simulink model "power_FCHPS_MEA2"  (R2017b)
settings: Solver=ode23tb  StartTime=0.0  StopTime=350  RelTol=1e-3  EnableMultiTasking=on
PreLoadFcn:
  | Ts=100e-6;
InitFcn:
  | Ts=100e-6;
undefined symbols (not defined in the file): DiscIntNeverNeededParam, Ion, Lithium
libraries: powerlib x94, simulink x8, powerlib_meascontrol x3, electricdrivelib x3
(part 1 of 4)
settings Model: SimulationMode=accelerator  Creator=MathWorks  LastModifiedBy=vv
settings DataIOCC: LimitDataPoints=on  SaveFormat=Array  SignalLoggingSaveFormat=ModelDataLogs
settings OptimizationCC: ExpressionDepthLimit=2147483647  EfficientMapNaN2IntZero=off  LifeSpan=inf
settings DebuggingCC: UnderspecifiedInitializationDetection=Classic  MergeDetectMultiDrivingBlocksExec=none  SolverPrmCheckMsg=warning  FcnCallInpInsideContextMsg=warning  AllowSymbolicDim=off  StateNameClashWarn=warning  SFUnexpectedBacktrackingDiag=warning  SFNoUnconditionalDefaultTransitionDiag=warning  SFExecutionAtInitializationDiag=none
settings HardwareCC: ProdBitPerPointer=32  ProdBitPerSizeT=32  ProdBitPerPtrDiffT=32  ProdLargestAtomicFloat=None  ProdIntDivRoundTo=Undefined  ProdEndianess=Unspecified  ProdWordSize=32  ProdHWDeviceType=32-bit Generic  TargetBitPerPointer=64  TargetBitPerSizeT=64  TargetBitPerPtrDiffT=64  TargetLongLongMode=on  TargetIntDivRoundTo=Zero  TargetEndianess=LittleEndian  TargetWordSize=64  TargetHWDeviceType=MATLAB Host  ProdEqTarget=off
settings ModelReferenceCC: PropagateSignalLabelsOutOfModel=off
settings CodeAppCC: MaxIdLength=128  StateflowObjectComments=on
settings GRTTargetCC: TargetLangStandard=C89/C90 (ANSI)  CombineOutputUpdateFcns=off  GRTInterface=on
settings ConfigComp: CovMetricSettings=dw  CovHtmlReporting=on  CovSaveCumulativeToWorkspaceVar=on  CovSaveSingleToWorkspaceVar=on  CovExternalEMLEnable=off  CovSFcnEnable=off
settings SimscapeCC: SimscapeNormalizeSystem=off

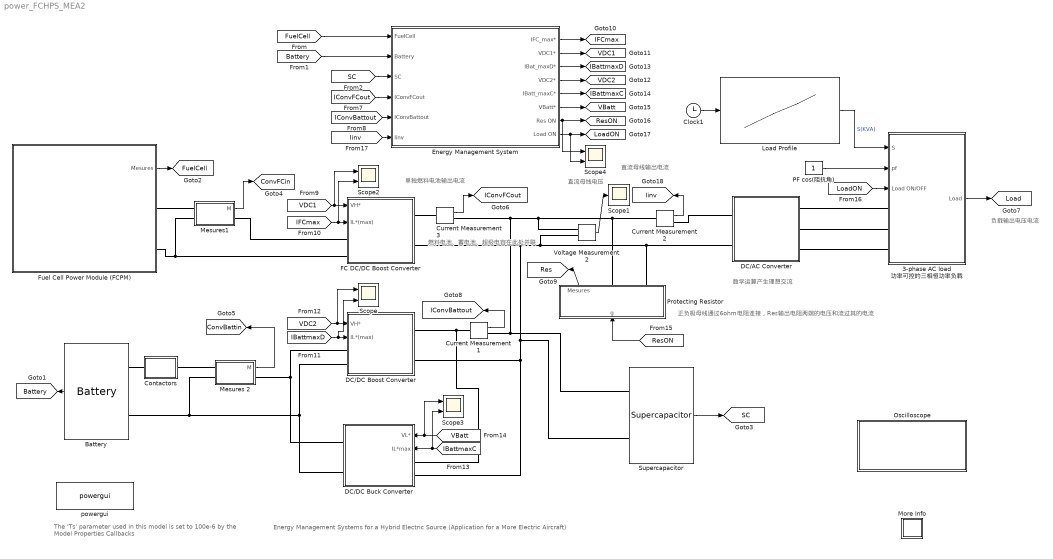
== system power_FCHPS_MEA2 ==
  note: 直流母线电压
  note: 直流母线输出电流
  note: 单独燃料电池输出电流
  note: 燃料电池、蓄电池、超级电容在此处并联
  note: 正负极母线通过6ohm电阻连接，Res输出电阻两端的电压和流过其的电流
  note: 数学运算产生理想交流
  note: 负载输出电压电流
  note: Energy Management Systems for a Hybrid Electric Source (Application for a More Electric Aircraft)
  note: The 'Ts' parameter used in this model
      | is set to 100e-6  by the Model Properties Callbacks
  3-phase AC load 功率可控的三相恒功率负载 : Subsystem
      mask Display: image(imread('load.png'))
  Battery : electricdrivelib/Extra Sources/Battery  BatType=Lithium-Ion  ShowTempParam=off  ThermalPreset=no  ShowAgeParam=off  NomV=48  NomQ=40  SOC=65  Batt_Tr=20  PresetModel=off  MaxQ=40  MinV=36  FullV=55.8714  Dis_rate=17.3913  R=0.012  Normal_OP=36.1739  expZone="[52.3         1.96]"  current=[20 80]  Units=Ampere-hour  Tci=20  NomT=20  T2=-30  MaxQ2=4.8  FullV2=7.1  Normal_OP2=5.72  expZone2="[6.58  1]"  Rca=0.6  ti=1000  Dp=0  Neq0=0  Tsim=1e6  Ta1=25  Qeol=5.4*0.9  Reol=0.013333*1.2  Char_age=[2.3478, 3]  Dis_age=[2.3478, 10]  N1=1500  N2=10500  N3=1000  N4=1400  Ta2=45  N5=950
  Clock1 : Clock
  Contactors : Subsystem
  Current Measurement1 : powerlib/Measurements/Current Measurement  PhasorSimulation=off  OutputType=Complex  PSBequivalent=0
  Current Measurement2 : powerlib/Measurements/Current Measurement  PhasorSimulation=off  OutputType=Complex  PSBequivalent=0
  Current Measurement3 : powerlib/Measurements/Current Measurement  PhasorSimulation=off  OutputType=Complex  PSBequivalent=0
  DC/AC Converter : Subsystem  mask(Average-value Inverter model){VL=200, f=400, n=97}
      mask prompts: VL "Output Line Voltage (Vrms)"; f "Output frequency (Hz)"; n "Nominal Efficiency (%)"
      mask help: This block represents an average-value inverter model which includes the converter efficiency.
      mask Display: image(imread('DCAC.bmp'))
  DC/DC Boost Converter : Subsystem  mask(Average value DC/DC boost converter){Inom=18, n=[80 88], Tr=0.1, CL=15.6}
      mask prompts: Inom "Full load current (A)"; n "Efficiency @ Full and 10% load  (%) [n1, n2]"; Tr "Response time (s) (Voltage Regulator)"; CL "Load Capacitance (F)"
      mask help: This block implements an average-value DC/DC boost converter. Two inputs are provided for output voltage regulation and input current limitation
      mask Display: image(imread('DCDC.bmp'))
  DC/DC Buck Converter : Subsystem  mask(Average Value Buck DC/DC Converter){Inom=20, n=[80 88], Tr=0.1, CL=100e-3}
      mask prompts: Inom "Full load current (A)"; n "Efficiency @ Full and 10% load (%) [n1, n2]"; Tr "Response Time (s) (Voltage Regulator)"; CL "Load Capacitance (F)"
      mask help: This block implements an average-value DC/DC buck converter. Two inputs are provided for output voltage regulation and output current limitation
      mask init:
      | L=10e-3; C=800e-6+CL;
      | thau_s=Tr;  %response time
      | %Current regulator
      | zetai=0.995;
      | thau_si=0.1/10; 
      | %zetawni=4.6/thau_si;
      | zetawni=(-log(0.05*sqrt(1-zetai^2)))/thau_si;
      | Kpi=2*L*zetawni;
      | wni=zetawni/zetai;
      | Kii=L*wni^2;
      | %Voltage regulator
      | zetav=0.995;
      | thau_sv=thau_s; %response time
      | %zetawnv=4.6/thau_sv;
      | zetawnv=(-log(0.05*sqrt(1-zetav^2)))/thau_sv;
      | Kpv=2*C*zetawnv;
      | wnv=zetawnv/zetav;
      | Kiv=C*wnv^2;
      | k=((n(1)/100)-(n(2)/100))/(Inom-(0.1*Inom));
      | k0=(n(1)/100)-k*Inom;
      mask DialogControl ParameterTabVar0 Prompt: Parameters
      mask Display: image(imread('DCDC.bmp'))
  Energy Management System : Subsystem  mask(Energy Management System){ems=State Machine Control Strategy}
      mask prompts: ems "Strategy:"
      mask help:
      | This block implements six types of energy management strategies, commonly used in Fuel Cell Hybrid Power Systems
      |
      | The ECMS and EEMS Control Strategies require the Optimization toolbox. The State Machine Control Strategy is selected automatically when the toolbox is not available.
      mask init:
      | [X1,X1m,X2,X2m,X3,X4,Y1,Y1m,Y2,Y2m,Y3,Y4,color1,color2]=spsdrivelogo;
      | 
      | SimulinkModel  = [gcs,'/Energy Management System'];
      | SimulinkModel2 = [gcs,'/Energy Management System/Model'];
      | 
      | switch ems
      |     case 'State Machine Control Strategy'
      |         set_param(SimulinkModel2,'OverrideUsingVariant','FrequencyDecoupling');
      |         
      |     case 'Classical PI Control Strategy'
      |         set_param(SimulinkModel2,'OverrideUsingVariant','ClassicalPI');
      |         
      |     case 'Rule Based Fuzzy Logic Control Strategy'
      |         if isempty(ver('fuzzy'))
      |             set_param(SimulinkModel,'ems','State Machine Control Strategy');
      |             set_param(SimulinkModel2,'OverrideUsingVariant','FrequencyDecoupling');
      |         else
      |             fuzzy_control=READFIS('fuzzy control.fis');
      |             set_param(SimulinkModel2,'OverrideUsingVariant','RuleBasedFuzzyLogic');
      |         end
      |         
      |     case 'Frequency Decoupling and State Machine Control Strategy'
      |         set_param(SimulinkModel2,'OverrideUsingVariant','FrequencyDecoupling');
      | 
      |     case 'Equivalent Consumption Minimization Strategy (ECMS)'
      |         if isempty(ver('optim'))
      |             set_param(SimulinkModel,'ems','State Machine Control Strategy');
      |             set_param(SimulinkModel2,'OverrideUsingVariant','FrequencyDecoupling');
      |         else
      |             set_param(SimulinkModel2,'OverrideUsingVariant','ECMS');
      |         end
      |         
      |     case 'External Energy Maximization Strategy (EEMS)'
      |         if isempty(ver('optim'))
      |             set_param(SimulinkModel,'ems','State Machine Control Strategy');
      |             set_param(SimulinkModel2,'OverrideUsingVariant','FrequencyDecoupling');
      |         else
      |             set_param(SimulinkModel2,'OverrideUsingVariant','EEMS');
      |         end
      | end
      mask TypeOptions ems: State Machine Control Strategy | Classical PI Control Strategy | Frequency Decoupling and State Machine Control Strategy | Equivalent Consumption Minimization Strategy (ECMS) | External Energy Maximization Strategy (EEMS)
      mask Display:
      | patch([X1 X1m],[Y1 Y1m],color1);
      | patch(X3,Y3,color2);
      | plot([X1 X1m X2 X2m X3 X4],[Y1 Y1m Y2 Y2m Y3 Y4]);
  FC DC/DC Boost Converter : Subsystem  mask(Average value DC/DC boost converter){Inom=45, n=[85 90], Tr=0.1, CL=15.6}
      mask prompts: Inom "Full load current (A)"; n "Efficiency @ Full and 10% load  (%) [n1, n2]"; Tr "Response time (s) (Voltage Regulator)"; CL "Load Capacitance (F)"
      mask help: This block implements an average-value DC/DC boost converter. Two inputs are provided for output voltage regulation and input current limitation
      mask Display: image(imread('DCDC.bmp'))
  Fuel Cell Power Module (FCPM) : Subsystem
      mask Display: image(imread('power_stack.bmp'))
  Load Profile : Lookup_n-D  NumberOfTableDimensions=1  BreakpointsForDimension1="[0    20    30    35    40    45    50    60    70    90   125   130   140   160   170   180   190 210   220   230   235   245   250   260   270   300   310   320   330   340     350]"  BreakpointsForDimension2=[0 571.55 685.8 800.15 914.4 1028.8 1143.1 1257.4 1371.7 1486 1600.3 1714.6 1828.9 1943.2 2057.5 2171.8 2286.1 2400.5 2514.7 2629.1 2743.3 2857.7 2971.9 3086.3 3200.5 3314.9 3429.2]  Table="[0         0         0         0         0    5.8000    4.8000    4.8000   10.0000    9.4000  10.5000    5.0000    8.8000    7.0000    7.3000    2.5000    8.5000    7.5000    9.0000    8.9000 8.7000    0.7000    2.9000    2.3500    2.9000    2.9000    2.4000    2.9000    2.9000         0     0]"  InternalRulePriority=Speed  RndMeth=Simplest  InputSameDT=on
  Mesures 2 : Subsystem
  Mesures1 : Subsystem
  More Info : Subsystem
      settings: OpenFcn=showdemo(bdroot(gcb))
      mask Display: disp('?')
  Oscilloscope : Subsystem
      mask Display: color('blue');disp('Measurements')
  PF cos(阻抗角) : Constant
  Protecting Resistor : Subsystem
      mask Display: image(imread('Res.jpg'))
  Scope{,2..4} (4 alike) : Scope  NumInputPorts=2
  Scope1 : Scope
  Supercapacitor : electricdrivelib/Extra Sources/Supercapacitor  C=15.6  Rdc=150e-3  Voltage=291.6  Ns=108  Np=1  Vinit=270  Temp=25  PresetModel=on  EstParam=off  Nc=1  r=1e-9  epsilon=6.0208e-10  Ich=10  Vstern="[0.161  2.7  7.8]"  Self_dis=on  Ioc=10  Vself="[48  47.8  47.06  44.65]"  demandeplot=off  I="[10  20 100  500]"  Units=sec  Vmax=0  If=0  deltaV=0.3  alpha=0.3  sec=0
      settings: SourceProductName=Simscape Power Systems  SourceProductBaseCode=PS
  Voltage Measurement2 : powerlib/Measurements/Voltage Measurement  PhasorSimulation=off  OutputType=Complex  PSBequivalent=0
  powergui : powerlib/powergui  Priority=1  SimulationMode=Discrete  SampleTime=Ts  frequency=60  Iterations=50  frequencyindice=0  Pbase=100e6  ErrMax=1e-4  UnitsV=kV  UnitsW=MW  buscounter=0  FunctionMessages=off  echomessages=off  EnableUseOfTLC=off  CurrentSourceSwitches=off  DisableSnubberDevices=off  DisableRonSwitches=off  DisableVfSwitches=off  DisplayEquations=off  SolverType=Tustin/Backward Euler (TBE)  Interpol=off  ExternalGateDelay=off  methode=off  Ts=0  x0status=blocks  SPID=off  SwTol=0  HookPort=off  RestoreLinks=warning  ResistiveCurrentMeasurement=off  Frange=[0:2:500]  Ylog=off  Xlog=on  ShowGrid=off  save=off  variable=ZData  structure=0  ZoomFFT=off  StartTime=0.0  cycles=1  DisplayStyle=1  fundamental=60  FreqAxis=off  MaxFrequency=1000  frequencyindicesteady=1  RmsSteady=1  display=off
  tag scope: Battery=global, ConvBattin=global, ConvFCin=global, FuelCell=global, IBattmaxC=global, IBattmaxD=global, IConvBattout=global, IConvFCout=global, IFCmax=global, Iinv=global, Load=global, LoadON=global, Res=global, ResON=global, SC=global, VBatt=global, VDC1=global, VDC2=global
  wires:
  Fuel Cell Power Module (FCPM)/1(Mesures) -> [FuelCell]
  Mesures1/1(M) -> [ConvFCin]
  Current Measurement1/1 -> [IConvBattout]
  Current Measurement3/1 -> [IConvFCout]
  Mesures 2/1(M) -> [ConvBattin]
  [FuelCell] -> Energy Management System/1(FuelCell)
  [Battery] -> Energy Management System/2(Battery)
  [SC] -> Energy Management System/3(SC)
  [IConvFCout] -> Energy Management System/4(IConvFCout)
  [IConvBattout] -> Energy Management System/5(IConvBattout)
  Energy Management System/1(IFC_max*) -> [IFCmax]
  Energy Management System/2(VDC1*) -> [VDC1]
  Energy Management System/3(IBat_maxD*) -> [IBattmaxD]
  Energy Management System/4(VDC2*) -> [VDC2]
  Energy Management System/5(IBatt_maxC*) -> [IBattmaxC]
  Energy Management System/6(VBatt*) -> [VBatt]
  Energy Management System/7(Res ON) -> Scope4/1, [ResON]
  Energy Management System/8(Load ON) -> Scope4/2, [LoadON]
  [VDC1] -> Scope2/1, FC DC/DC Boost Converter/1(VH*)
  [IFCmax] -> Scope2/2, FC DC/DC Boost Converter/2(IL*(max))
  [VDC2] -> Scope/1, DC/DC Boost Converter/1(VH*)
  [IBattmaxD] -> Scope/2, DC/DC Boost Converter/2(IL*(max))
  [VBatt] -> Scope3/1, DC/DC Buck Converter/1(VL*)
  Current Measurement2/1 -> [Iinv]
  [Iinv] -> Energy Management System/6(Iinv)
  [ResON] -> Protecting Resistor/1(g)
  Protecting Resistor/1(Mesures) -> [Res]
  Clock1/1 -> Load Profile/1
  [LoadON] -> 3-phase AC load 功率可控的三相恒功率负载/3(Load ON/OFF)
  PF cos(阻抗角)/1 -> 3-phase AC load 功率可控的三相恒功率负载/2(pf)
  3-phase AC load 功率可控的三相恒功率负载/1(Load) -> [Load]
  Load Profile/1 -> 3-phase AC load 功率可控的三相恒功率负载/1(S)  "S(KVA)"
  Battery/1 -> [Battery]
  Supercapacitor/1 -> [SC]
  Voltage Measurement2/1 -> Scope1/1
  [IBattmaxC] -> Scope3/2, DC/DC Buck Converter/2(IL*max)
  connections:
  DC/DC Buck Converter/RConn2 -- DC/DC Boost Converter/LConn2 -- Mesures 2/LConn2 -- Battery/LConn2
  Fuel Cell Power Module (FCPM)/RConn1 -- Mesures1/LConn1
  DC/DC Buck Converter/LConn1 -- Current Measurement1/LConn1 -- DC/DC Boost Converter/RConn1
  FC DC/DC Boost Converter/RConn1 -- Current Measurement3/LConn1
  DC/AC Converter/RConn1 -- 3-phase AC load 功率可控的三相恒功率负载/LConn1
  DC/AC Converter/RConn2 -- 3-phase AC load 功率可控的三相恒功率负载/LConn2
  DC/AC Converter/RConn3 -- 3-phase AC load 功率可控的三相恒功率负载/LConn3
  Contactors/RConn1 -- Mesures 2/LConn1
  Mesures1/RConn1 -- FC DC/DC Boost Converter/LConn1
  FC DC/DC Boost Converter/LConn2 -- Mesures1/LConn2 -- Fuel Cell Power Module (FCPM)/RConn2
  DC/DC Buck Converter/RConn1 -- DC/DC Boost Converter/LConn1 -- Mesures 2/RConn1
  Current Measurement2/RConn1 -- DC/AC Converter/LConn1
  Supercapacitor/LConn1 -- Current Measurement3/RConn1 -- Voltage Measurement2/LConn1 -- Current Measurement2/LConn1 -- Protecting Resistor/RConn1 -- Current Measurement1/RConn1
  DC/DC Buck Converter/LConn2 -- DC/DC Boost Converter/RConn2 -- Supercapacitor/LConn2 -- Voltage Measurement2/LConn2 -- Protecting Resistor/RConn2 -- DC/AC Converter/LConn2 -- FC DC/DC Boost Converter/RConn2
  Battery/LConn1 -- Contactors/LConn1

== system power_FCHPS_MEA2/3-phase AC load 功率可控的三相恒功率负载 ==
  S : Inport
  pf : Inport  Port=2
  Load ON/OFF : Inport  Port=3
  1 kW 0.5 kvar @ 208V3 : powerlib/Elements/Three-Phase Parallel RLC Load  LConnTagsString=A|B|C  Configuration=Y (grounded)  NominalVoltage=200  Vabc=[1e3 1e3 1e3]  Vabcp=[1e3 1e3 1e3]  NominalFrequency=400  UnbalancedPower=off  ActivePower=1e-6  InductivePower=0  CapacitivePower=0  Pabc=[10e3 9e3 11e3]  QLabc=[100 90 110]  QCabc=[100 90 110]  Pabcp=[10e3 9e3 11e3]  QLabcp=[100 90 110]  QCabcp=[100 90 110]  Measurements=None  LoadType=constant Z
  Complex to Real-Imag : ComplexToRealImag
  Controlled Current Source : powerlib/Electrical Sources/Controlled Current Source  Initialize=off  Source_Type=AC  Amplitude=0  Phase=0  Frequency=0  Measurements=None
  Controlled Current Source1 : powerlib/Electrical Sources/Controlled Current Source  Initialize=off  Source_Type=AC  Amplitude=0  Phase=0  Frequency=0  Measurements=None
  Demux : Demux  Outputs=3
  Demux1 : Demux  Outputs=2
  Divide2 : Product  Inputs=/*
  Dynamic Impedance : Subsystem
  Gain : Gain  Gain=1/3
  Ground : Ground
  Mux1 : Mux  Inputs=3
  Mux2 : Mux  Inputs=2
  PLL (3ph) : powerlib_meascontrol/PLL/PLL (3ph)  Fmin=390  Par_Init=[0, 60]  ParK=[180, 3200, 1]  TcD=1e-4  MaxRateChangeFreq=12  FilterCutOffFreq=25  Ts=0  AGC=on
  Product : Product  RndMeth=Zero
  Real-Imag to Complex : RealImagToComplex
  Saturation : Saturate  UpperLimit=1  LowerLimit=0.001
  Saturation1 : Saturate  UpperLimit=1  LowerLimit=-1
  Saturation2 : Saturate  UpperLimit=inf  LowerLimit=0.001
  Selector : Selector  InputPortWidth=3  IndexOptions=Index vector (dialog)  Indices=[1 2]  OutputSizes=1
  Terminator1 : Terminator
  Terminator2 : Terminator
  Three-Phase V-I Measurement1 : powerlib/Measurements/Three-Phase V-I Measurement  VoltageMeasurement=phase-to-ground  SetLabelV=off  LabelV=Vabc  Vpu=off  VpuLL=off  CurrentMeasurement=yes  SetLabelI=off  LabelI=Iabc  Ipu=off  Pbase=100e6  Vbase=500e3  OutputType=Complex  PhasorSimulation=off  PSBequivalent=0
  Unit Delay : UnitDelay  SampleTime=Ts
  Unit Delay1 : UnitDelay  SampleTime=Ts
  abc to dq0 : powerlib_meascontrol/Transformations/abc to dq0  Alignment=90 degrees behind phase A axis
  dq0 to abc : powerlib_meascontrol/Transformations/dq0 to abc  Alignment=90 degrees behind phase A axis
  A : PMIOPort  Port=1  Side=Left
  B : PMIOPort  Port=2  Side=Left
  C : PMIOPort  Port=3  Side=Left
  Load : Outport
  wires:
  Divide2/1 -> Complex to Real-Imag/1
  Dynamic Impedance/1(Z) -> Divide2/1
  Three-Phase V-I Measurement1/1 -> PLL (3ph)/1, abc to dq0/1, Mux2/1
  Demux/3 -> Terminator1/1
  Mux1/1 -> dq0 to abc/1
  Ground/1 -> Mux1/3
  Complex to Real-Imag/2 -> Mux1/2
  Complex to Real-Imag/1 -> Mux1/1
  Real-Imag to Complex/1 -> Divide2/2
  Demux/2 -> Real-Imag to Complex/2
  Demux/1 -> Real-Imag to Complex/1
  S/1 -> Saturation2/1
  Selector/1 -> Demux1/1
  Demux1/1 -> Unit Delay/1
  Demux1/2 -> Unit Delay1/1
  pf/1 -> Saturation1/1
  Gain/1 -> Dynamic Impedance/1(S)
  Unit Delay/1 -> Controlled Current Source/1
  Unit Delay1/1 -> Controlled Current Source1/1
  Three-Phase V-I Measurement1/2 -> Mux2/2
  Mux2/1 -> Load/1
  Saturation/1 -> Product/2
  Load ON/OFF/1 -> Saturation/1
  Product/1 -> Gain/1
  Saturation1/1 -> Dynamic Impedance/2(pf)
  Saturation2/1 -> Product/1
  PLL (3ph)/2 -> abc to dq0/2, dq0 to abc/2
  abc to dq0/1 -> Demux/1
  PLL (3ph)/1 -> Terminator2/1
  dq0 to abc/1 -> Selector/1
  connections:
  C/RConn1 -- Three-Phase V-I Measurement1/LConn3 -- 1 kW 0.5 kvar @ 208V3/LConn3
  Three-Phase V-I Measurement1/LConn2 -- B/RConn1 -- 1 kW 0.5 kvar @ 208V3/LConn2
  Three-Phase V-I Measurement1/LConn1 -- A/RConn1 -- 1 kW 0.5 kvar @ 208V3/LConn1
  Controlled Current Source1/LConn1 -- Three-Phase V-I Measurement1/RConn2
  Controlled Current Source/RConn1 -- Three-Phase V-I Measurement1/RConn3 -- Controlled Current Source1/RConn1
  Controlled Current Source/LConn1 -- Three-Phase V-I Measurement1/RConn1

== system power_FCHPS_MEA2/Contactors ==
  Compare To Zero : simulink/Logic and Bit Operations/Compare To Zero  relop=>  OutDataTypeStr=boolean
  Current Measurement : powerlib/Measurements/Current Measurement  PhasorSimulation=off  OutputType=Complex  PSBequivalent=0
  Ideal Switch : powerlib/Power Electronics/Ideal Switch  Ron=0.001  Lon=0  IC=0  Rs=1e5  Cs=inf  Measurements=off
  Series RLC Branch : powerlib/Elements/Series RLC Branch  LConnTagsString=__new0  RConnTagsString=__new0  BranchType=R  Resistance=0.175  Inductance=1e-3  SetiL0=off  InitialCurrent=0  Capacitance=1e-6  Setx0=off  InitialVoltage=0  Measurements=None
  Series RLC Branch1 : powerlib/Elements/Series RLC Branch  LConnTagsString=__new0  RConnTagsString=__new0  BranchType=R  Resistance=0.07  Inductance=1e-3  SetiL0=off  InitialCurrent=0  Capacitance=1e-6  Setx0=off  InitialVoltage=0  Measurements=None
  A : PMIOPort  Port=1  Side=Left
  B : PMIOPort  Port=2  Side=Right
  wires:
  Current Measurement/1 -> Compare To Zero/1
  Compare To Zero/1 -> Ideal Switch/1
  connections:
  Ideal Switch/LConn1 -- Series RLC Branch/LConn1 -- Current Measurement/RConn1
  A/RConn1 -- Current Measurement/LConn1
  Ideal Switch/RConn1 -- Series RLC Branch1/LConn1
  Series RLC Branch1/RConn1 -- B/RConn1 -- Series RLC Branch/RConn1

== system power_FCHPS_MEA2/DC//AC Converter ==
  note: Ubc*Ic
  note: Ia*Uab
  Add : Sum  Inputs=+-
  Control open loop1 : Subsystem
  Controlled Current Source : powerlib/Electrical Sources/Controlled Current Source  Initialize=on  Source_Type=AC  Amplitude=0  Phase=0  Frequency=0  Measurements=None
  Controlled Voltage Source : powerlib/Electrical Sources/Controlled Voltage Source  Initialize=on  Source_Type=AC  Amplitude=0  Phase=0  Frequency=0  Measurements=None
  Controlled Voltage Source1 : powerlib/Electrical Sources/Controlled Voltage Source  Initialize=on  Source_Type=AC  Amplitude=0  Phase=0  Frequency=0  Measurements=None
  Current Measurement : powerlib/Measurements/Current Measurement  PhasorSimulation=off  OutputType=Complex  PSBequivalent=0
  Current Measurement2 : powerlib/Measurements/Current Measurement  PhasorSimulation=off  OutputType=Complex  PSBequivalent=0
  Divide : Product  Inputs=*/
  Gain1 : Gain  Gain=n/100
  Product : Product  RndMeth=Zero
  Product1 : Product  RndMeth=Zero
  Saturation : Saturate  UpperLimit=inf  LowerLimit=0.01
  Selector : Selector  InputPortWidth=3  IndexOptions=Index vector (dialog)  Indices=1  OutputSizes=1
  Selector1 : Selector  InputPortWidth=3  IndexOptions=Index vector (dialog)  Indices=2  OutputSizes=1
  Unit Delay : UnitDelay  SampleTime=Ts
  Vab-inv1 : powerlib/Measurements/Voltage Measurement  Tag=PoWeRsYsTeMmEaSuReMeNt  PhasorSimulation=off  OutputType=Magnitude  PSBequivalent=0
  Vab-inv2 : powerlib/Measurements/Voltage Measurement  Tag=PoWeRsYsTeMmEaSuReMeNt  PhasorSimulation=off  OutputType=Magnitude  PSBequivalent=0
  Vab-inv4 : powerlib/Measurements/Voltage Measurement  Tag=PoWeRsYsTeMmEaSuReMeNt  PhasorSimulation=off  OutputType=Magnitude  PSBequivalent=0
  A : PMIOPort  Port=1  Side=Right
  +Vdc : PMIOPort  Port=2  Side=Left
  B : PMIOPort  Port=3  Side=Right
  -Vdc : PMIOPort  Port=4  Side=Left
  C : PMIOPort  Port=5  Side=Right
  wires:
  Vab-inv1/1 -> Product/2
  Current Measurement/1 -> Product/1
  Product/1 -> Add/1
  Vab-inv2/1 -> Product1/1
  Current Measurement2/1 -> Product1/2
  Product1/1 -> Add/2
  Add/1 -> Divide/1
  Vab-inv4/1 -> Gain1/1
  Saturation/1 -> Divide/2
  Divide/1 -> Unit Delay/1
  Control open loop1/1(g) -> Selector/1, Selector1/1
  Selector/1 -> Controlled Voltage Source/1
  Selector1/1 -> Controlled Voltage Source1/1
  Gain1/1 -> Saturation/1
  Unit Delay/1 -> Controlled Current Source/1
  connections:
  -Vdc/RConn1 -- Vab-inv4/LConn2 -- Controlled Current Source/RConn1
  Controlled Voltage Source/LConn1 -- Controlled Voltage Source1/RConn1 -- Vab-inv1/LConn2 -- Vab-inv2/LConn1 -- B/RConn1
  Controlled Voltage Source/RConn1 -- Vab-inv1/LConn1 -- Current Measurement/LConn1
  Controlled Voltage Source1/LConn1 -- Vab-inv2/LConn2 -- Current Measurement2/LConn1
  A/RConn1 -- Current Measurement/RConn1
  C/RConn1 -- Current Measurement2/RConn1
  +Vdc/RConn1 -- Controlled Current Source/LConn1 -- Vab-inv4/LConn1

== system power_FCHPS_MEA2/DC//DC Boost Converter ==
  VH* : Inport
  IL*(max) : Inport  Port=2
  Constant : Constant  Value=60
  DC/DC Boost Converter : Subsystem  mask(Average Value Boost DC/DC Converter){Inom=Inom, n=n, Tr=Tr, CL=CL}
      mask prompts: Inom "Full load current (A)"; n "Efficiency at Full and 10% load (%) [n1, n2]"; Tr "Response Time (s) (Voltage Regulator)"; CL "Load Capacitance (F)"
      mask help: This block implements an average-value DC/DC boost converter. Two inputs are provided for output voltage regulation and input current limitation
      mask init:
      | L=100e-6; C=800e-6+CL;
      | thau_s=Tr;  % response time
      | %Current regulator
      | zetai=0.707;
      | thau_si=0.1/10; 
      | %zetawni=4.6/thau_si;
      | zetawni=(-log(0.05*sqrt(1-zetai^2)))/thau_si;
      | Kpi=2*L*zetawni;
      | wni=zetawni/zetai;
      | Kii=L*wni^2;
      | %Voltage regulator
      | zetav=0.707;
      | thau_sv=thau_s; %response time
      | %zetawnv=4.6/thau_sv;
      | zetawnv=(-log(0.05*sqrt(1-zetav^2)))/thau_sv;
      | Kpv=2*C*zetawnv;
      | wnv=zetawnv/zetav;
      | Kiv=C*wnv^2;
      | k=((n(1)/100)-(n(2)/100))/(Inom-(0.1*Inom));
      | k0=(n(1)/100)-k*Inom;
  DC/DC Buck Converter For DC bus precharge : Subsystem  mask(Average Value Buck DC/DC Converter){Inom=0.88*Inom, n=n, Tr=Tr, CL=CL}
      mask prompts: Inom "Full oad current (A)"; n "Efficiency @ Full and 10% load (%) [n1, n2]"; Tr "Response Time (s) (Voltage Regulator)"; CL "Load Capacitance (F)"
      mask help: This block implements an average-value DC/DC buck converter. Two inputs are provided for output voltage regulation and output current limitation
      mask init:
      | L=100e-6; C=800e-6+CL;
      | thau_s=Tr;  %response time
      | %Current regulator
      | zetai=0.707;
      | thau_si=0.1/10; 
      | %zetawni=4.6/thau_si;
      | zetawni=(-log(0.05*sqrt(1-zetai^2)))/thau_si;
      | Kpi=2*L*zetawni;
      | wni=zetawni/zetai;
      | Kii=L*wni^2;
      | %Voltage regulator
      | zetav=0.707;
      | thau_sv=thau_s; %response time
      | %zetawnv=4.6/thau_sv;
      | zetawnv=(-log(0.05*sqrt(1-zetav^2)))/thau_sv;
      | Kpv=2*C*zetawnv;
      | wnv=zetawnv/zetav;
      | Kiv=C*wnv^2;
      | k=((n(1)/100)-(n(2)/100))/(Inom-(0.1*Inom));
      | k0=(n(1)/100)-k*Inom;
  +VH : PMIOPort  Port=1  Side=Right
  +VL : PMIOPort  Port=2  Side=Left
  -VH : PMIOPort  Port=3  Side=Right
  -VL : PMIOPort  Port=4  Side=Left
  wires:
  IL*(max)/1 -> DC/DC Boost Converter/2(IL*(max))
  VH*/1 -> DC/DC Boost Converter/1(VH*)
  Constant/1 -> DC/DC Buck Converter For DC bus precharge/1(VL*)
  DC/DC Buck Converter For DC bus precharge/1(Iinbuck) -> [Iinbuck]
  [Iinbuck] -> DC/DC Boost Converter/3(Iinbuck)
  connections:
  DC/DC Boost Converter/RConn1 -- +VH/RConn1 -- DC/DC Buck Converter For DC bus precharge/RConn1
  DC/DC Boost Converter/LConn1 -- +VL/RConn1 -- DC/DC Buck Converter For DC bus precharge/LConn1
  DC/DC Boost Converter/LConn2 -- -VL/RConn1 -- DC/DC Buck Converter For DC bus precharge/LConn2
  DC/DC Buck Converter For DC bus precharge/RConn2 -- -VH/RConn1 -- DC/DC Boost Converter/RConn2

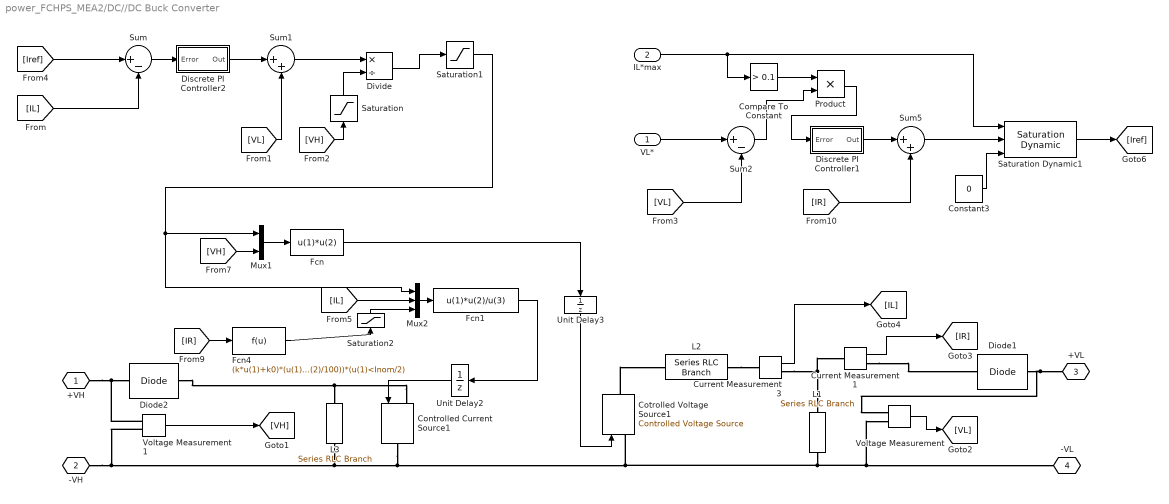
== system power_FCHPS_MEA2/DC//DC Buck Converter ==
  VL* : Inport
  IL*max : Inport  Port=2
  Compare To Constant : simulink/Logic and Bit Operations/Compare To Constant  relop=>  const=0.1  OutDataTypeStr=uint8
  Constant3 : Constant  Value=0
  Controlled Current Source1 : powerlib/Electrical Sources/Controlled Current Source  Initialize=on  Source_Type=DC  Amplitude=0  Phase=0  Frequency=0  Measurements=None
  Cotrolled Voltage Source1 : powerlib/Electrical Sources/Controlled Voltage Source  Initialize=on  Source_Type=DC  Amplitude=0  Phase=0  Frequency=0  Measurements=None
  Current Measurement1 : powerlib/Measurements/Current Measurement  PhasorSimulation=off  OutputType=Complex  PSBequivalent=0
  Current Measurement3 : powerlib/Measurements/Current Measurement  PhasorSimulation=off  OutputType=Complex  PSBequivalent=0
  Diode1 : powerlib/Power Electronics/Diode  Ron=0.001  Lon=0  Vf=0  IC=0  UseSnubber=off  Rs=1e6  Cs=250e-9  Measurements=off
  Diode2 : powerlib/Power Electronics/Diode  Ron=0.001  Lon=0  Vf=0  IC=0  UseSnubber=off  Rs=1e6  Cs=250e-9  Measurements=off
  Discrete PI Controller1 : Subsystem  DialogController=POWERSYS.PowerSysDialog  mask(Discrete PI Controller){Kp=Kpv, Ki=Kiv, Par_Limits=[1 -1], Init=0, Ts=Ts}
      mask prompts: Kp "Proportional gain (Kp):"; Ki "Integral gain (Ki):"; Par_Limits "Output limits: [ Upper   Lower ]"; Init "Output initial value:"; Ts "Sample time:"
      mask help: This block implements a discrete PI controller.
      mask init:
      | UpperLimit=Par_Limits(1);
      | LowerLimit=Par_Limits(2);
      | power_initmask();
      mask Help: This block is part of a subset of blocks in the Extras library that does not have documentation associated with it, other than the block mask description.
      mask Display: disp('PI');
  Discrete PI Controller2 : Subsystem  DialogController=POWERSYS.PowerSysDialog  mask(Discrete PI Controller){Kp=Kpi, Ki=Kii, Par_Limits=[1 -1], Init=0, Ts=Ts}
      mask prompts: Kp "Proportional gain (Kp):"; Ki "Integral gain (Ki):"; Par_Limits "Output limits: [ Upper   Lower ]"; Init "Output initial value:"; Ts "Sample time:"
      mask help: This block implements a discrete PI controller.
      mask init:
      | UpperLimit=Par_Limits(1);
      | LowerLimit=Par_Limits(2);
      | power_initmask();
      mask Help: This block is part of a subset of blocks in the Extras library that does not have documentation associated with it, other than the block mask description.
      mask Display: disp('PI');
  Divide : Product  Inputs=*/  SampleTime=Ts
  Fcn : Fcn  Expr=u(1)*u(2)
  Fcn1 : Fcn  Expr=u(1)*u(2)/u(3)
  Fcn4 : Fcn  Expr=(k*u(1)+k0)*(u(1)>=Inom/2)+((n(2)/100))*(u(1)<Inom/2)  SampleTime=Ts
  L1 : powerlib/Elements/Series RLC Branch  LConnTagsString=__new0  RConnTagsString=__new0  BranchType=RC  Resistance=0.01  Inductance=10e-6  SetiL0=off  InitialCurrent=100  Capacitance=800e-6  Setx0=off  InitialVoltage=0  Measurements=None
  L2 : powerlib/Elements/Series RLC Branch  LConnTagsString=__new0  RConnTagsString=__new0  BranchType=L  Resistance=0.3  Inductance=L  SetiL0=off  InitialCurrent=100  Capacitance=100e-6  Setx0=off  InitialVoltage=0  Measurements=None
  L3 : powerlib/Elements/Series RLC Branch  LConnTagsString=__new0  RConnTagsString=__new0  BranchType=R  Resistance=2e6  Inductance=10e-6  SetiL0=off  InitialCurrent=100  Capacitance=800e-6  Setx0=off  InitialVoltage=0  Measurements=None
  Mux1 : Mux  Inputs=2
  Mux2 : Mux  Inputs=3
  Product : Product  RndMeth=Zero
  Saturation : Saturate  UpperLimit=inf  LowerLimit=0.001  SampleTime=Ts
  Saturation Dynamic1 : simulink/Discontinuities/Saturation Dynamic  OutMin=[]  OutMax=[]  OutDataTypeStr=Inherit: Same as second input  OutDataType=fixdt(1, 16)  OutScaling=2^-10  DoSatur=off
  Saturation1 : Saturate  UpperLimit=1  LowerLimit=0  SampleTime=Ts
  Saturation2 : Saturate  UpperLimit=inf  LowerLimit=0.001  SampleTime=Ts
  Sum : Sum  Inputs=|+-
  Sum1 : Sum  Inputs=|++
  Sum2 : Sum  Inputs=|+-
  Sum5 : Sum  Inputs=|++
  Unit Delay2 : UnitDelay  SampleTime=Ts
  Unit Delay3 : UnitDelay  SampleTime=Ts
  Voltage Measurement : powerlib/Measurements/Voltage Measurement  PhasorSimulation=off  OutputType=Complex  PSBequivalent=0
  Voltage Measurement1 : powerlib/Measurements/Voltage Measurement  PhasorSimulation=off  OutputType=Complex  PSBequivalent=0
  +VH : PMIOPort  Tag=PMCPort  Port=1  Side=Left
  -VH : PMIOPort  Tag=PMCPort  Port=2  Side=Left
  +VL : PMIOPort  Tag=PMCPort  Port=3  Side=Right
  -VL : PMIOPort  Tag=PMCPort  Port=4  Side=Right
  wires:
  Mux2/1 -> Fcn1/1
  Mux1/1 -> Fcn/1
  Voltage Measurement/1 -> [VL]
  Voltage Measurement1/1 -> [VH]
  Current Measurement1/1 -> [IR]
  [IL] -> Mux2/2
  [VH] -> Mux1/2
  Fcn/1 -> Unit Delay3/1
  Fcn1/1 -> Unit Delay2/1
  [IL] -> Sum/2
  Sum/1 -> Discrete PI Controller2/1(Error)
  Discrete PI Controller2/1(Out) -> Sum1/1
  [VL] -> Sum1/2
  Sum1/1 -> Divide/1
  [VH] -> Saturation/1
  Saturation/1 -> Divide/2
  Divide/1 -> Saturation1/1
  Saturation1/1 -> Mux2/1, Mux1/1
  Sum2/1 -> Product/2
  Discrete PI Controller1/1(Out) -> Sum5/1
  Sum5/1 -> Saturation Dynamic1/2
  Constant3/1 -> Saturation Dynamic1/3
  Saturation Dynamic1/1 -> [Iref]
  Current Measurement3/1 -> [IL]
  [VL] -> Sum2/2
  [Iref] -> Sum/1
  IL*max/1 -> Saturation Dynamic1/1, Compare To Constant/1
  [IR] -> Fcn4/1
  VL*/1 -> Sum2/1
  Compare To Constant/1 -> Product/1
  Product/1 -> Discrete PI Controller1/1(Error)
  Saturation2/1 -> Mux2/3
  Fcn4/1 -> Saturation2/1
  [IR] -> Sum5/2
  Unit Delay2/1 -> Controlled Current Source1/1
  Unit Delay3/1 -> Cotrolled Voltage Source1/1
  connections:
  Voltage Measurement1/LConn2 -- -VH/RConn1 -- Cotrolled Voltage Source1/LConn1 -- -VL/RConn1 -- Voltage Measurement/LConn2 -- L1/RConn1 -- Controlled Current Source1/RConn1 -- L3/RConn1
  Voltage Measurement1/LConn1 -- Diode2/LConn1 -- +VH/RConn1
  Cotrolled Voltage Source1/RConn1 -- L2/RConn1
  Current Measurement3/RConn1 -- Current Measurement1/LConn1 -- L1/LConn1
  Current Measurement1/RConn1 -- Diode1/LConn1
  Diode1/RConn1 -- Voltage Measurement/LConn1 -- +VL/RConn1
  Controlled Current Source1/LConn1 -- Diode2/RConn1 -- L3/LConn1
  L2/LConn1 -- Current Measurement3/LConn1

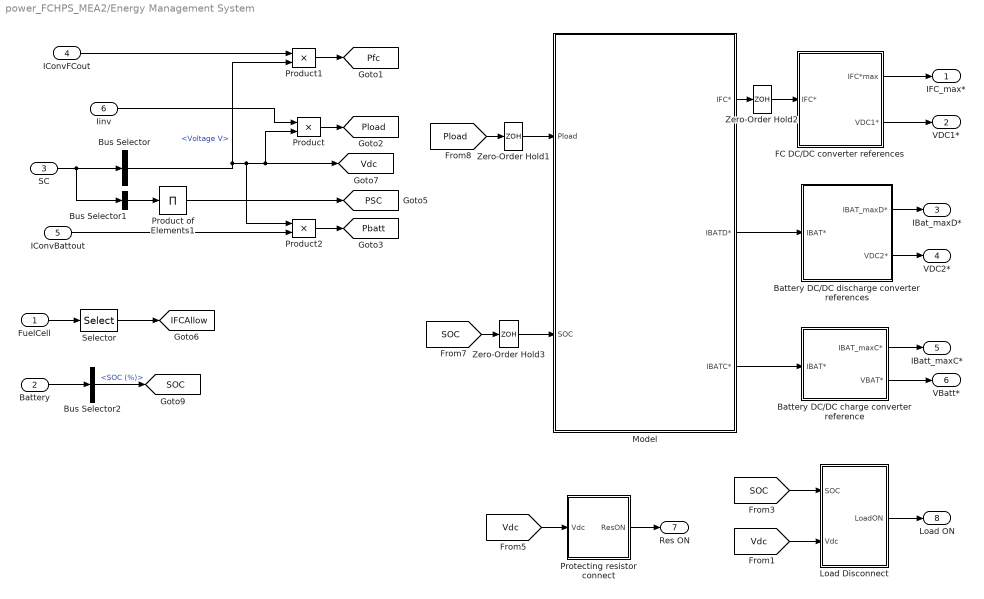
== system power_FCHPS_MEA2/Energy Management System ==
  FuelCell : Inport
  Battery : Inport  Port=2
  SC : Inport  Port=3
  IConvFCout : Inport  Port=4
  IConvBattout : Inport  Port=5
  Iinv : Inport  Port=6
  Battery DC/DC charge converter reference : Subsystem
  "Battery DC/DC discharge converter references " : Subsystem
  Bus Selector : BusSelector  OutputSignals=Voltage V
  Bus Selector1 : BusSelector  OutputSignals=Voltage V,Current I  OutputAsBus=on
  Bus Selector2 : BusSelector  OutputSignals=SOC (%)
  FC DC/DC converter references : Subsystem
  Load Disconnect : Subsystem
  Model : Subsystem  BlockChoice=State Machine Control  Variant=on  OverrideUsingVariant=FrequencyDecoupling
      settings: AttributesFormatString=%<BlockChoice>
  Product : Product  RndMeth=Zero
  Product of Elements1 : Product  Inputs=*
  Product1 : Product  RndMeth=Zero
  Product2 : Product  RndMeth=Zero
  Protecting resistor connect : Subsystem
  Selector : Selector  InputPortWidth=7  IndexOptions=Index vector (dialog)  Indices=1  OutputSizes=1
  Zero-Order Hold1 : ZeroOrderHold  SampleTime=200e-3
  Zero-Order Hold2 : ZeroOrderHold  SampleTime=200e-3
  Zero-Order Hold3 : ZeroOrderHold  SampleTime=200e-3
  IFC_max* : Outport
  VDC1* : Outport  Port=2
  IBat_maxD* : Outport  Port=3
  VDC2* : Outport  Port=4
  IBatt_maxC* : Outport  Port=5
  VBatt* : Outport  Port=6
  Res ON : Outport  Port=7
  Load ON : Outport  Port=8
  tag scope: IFCAllow=global, PSC=global, Pbatt=global, Pfc=global, Pload=global, SOC=global, Vdc=global
  wires:
  Bus Selector/1 -> Product1/2, Product2/1, Product/2, [Vdc]  "<Voltage V>"
  IConvFCout/1 -> Product1/1
  IConvBattout/1 -> Product2/2
  Iinv/1 -> Product/1
  SC/1 -> Bus Selector/1, Bus Selector1/1
  Product/1 -> [Pload]
  Product1/1 -> [Pfc]
  Product2/1 -> [Pbatt]
  Bus Selector1/1 -> Product of Elements1/1
  Product of Elements1/1 -> [PSC]
  FuelCell/1 -> Selector/1
  Selector/1 -> [IFCAllow]
  Battery/1 -> Bus Selector2/1
  Bus Selector2/1 -> [SOC]  "<SOC (%)>"
  [SOC] -> Load Disconnect/1(SOC)
  [Vdc] -> Load Disconnect/2(Vdc)
  Load Disconnect/1(LoadON) -> Load ON/1
  [Vdc] -> Protecting resistor connect/1(Vdc)
  Protecting resistor connect/1(ResON) -> Res ON/1
  Model/1(IFC*) -> Zero-Order Hold2/1
  FC DC/DC converter references/1(IFC*max) -> IFC_max*/1
  FC DC/DC converter references/2(VDC1*) -> VDC1*/1
  "Battery DC/DC discharge converter references "/1(IBAT_maxD*) -> IBat_maxD*/1
  "Battery DC/DC discharge converter references "/2(VDC2*) -> VDC2*/1
  Battery DC/DC charge converter reference/1(IBAT_maxC*) -> IBatt_maxC*/1
  Battery DC/DC charge converter reference/2(VBAT*) -> VBatt*/1
  [Pload] -> Zero-Order Hold1/1
  [SOC] -> Zero-Order Hold3/1
  Zero-Order Hold2/1 -> FC DC/DC converter references/1(IFC*)
  Model/2(IBATD*) -> "Battery DC/DC discharge converter references "/1(IBAT*)
  Model/3(IBATC*) -> Battery DC/DC charge converter reference/1(IBAT*)
  Zero-Order Hold1/1 -> Model/1(Pload)
  Zero-Order Hold3/1 -> Model/2(SOC)

== system power_FCHPS_MEA2/FC DC//DC Boost Converter ==
  VH* : Inport
  IL*(max) : Inport  Port=2
  Constant : Constant  Value=60
  DC/DC Boost Converter : Subsystem  mask(Average Value Boost DC/DC Converter){Inom=Inom, n=n, Tr=Tr, CL=CL}
      mask prompts: Inom "Full load current (A)"; n "Efficiency at Full and 10% load (%) [n1, n2]"; Tr "Response Time (s) (Voltage Regulator)"; CL "Load Capacitance (F)"
      mask help: This block implements an average-value DC/DC boost converter. Two inputs are provided for output voltage regulation and input current limitation
      mask init: same as power_FCHPS_MEA2/DC//DC Boost Converter/DC/DC Boost Converter
  DC/DC Buck Converter For DC bus precharge : Subsystem  mask(Average Value Buck DC/DC Converter){Inom=0.88*Inom, n=n, Tr=Tr, CL=CL}
      mask prompts: Inom "Full oad current (A)"; n "Efficiency @ Full and 10% load (%) [n1, n2]"; Tr "Response Time (s) (Voltage Regulator)"; CL "Load Capacitance (F)"
      mask help: This block implements an average-value DC/DC buck converter. Two inputs are provided for output voltage regulation and output current limitation
      mask init: same as power_FCHPS_MEA2/DC//DC Boost Converter/DC/DC Buck Converter For DC bus precharge
  +VH : PMIOPort  Port=1  Side=Right
  +VL : PMIOPort  Port=2  Side=Left
  -VH : PMIOPort  Port=3  Side=Right
  -VL : PMIOPort  Port=4  Side=Left
  wires:
  [Iinbuck] -> DC/DC Boost Converter/3(Iinbuck)
  DC/DC Buck Converter For DC bus precharge/1(Iinbuck) -> [Iinbuck]
  Constant/1 -> DC/DC Buck Converter For DC bus precharge/1(VL*)
  VH*/1 -> DC/DC Boost Converter/1(VH*)
  IL*(max)/1 -> DC/DC Boost Converter/2(IL*(max)), DC/DC Buck Converter For DC bus precharge/2(IH*(max))
  connections:
  DC/DC Boost Converter/RConn2 -- -VH/RConn1 -- DC/DC Buck Converter For DC bus precharge/RConn2
  DC/DC Buck Converter For DC bus precharge/LConn2 -- -VL/RConn1 -- DC/DC Boost Converter/LConn2
  DC/DC Buck Converter For DC bus precharge/LConn1 -- +VL/RConn1 -- DC/DC Boost Converter/LConn1
  DC/DC Buck Converter For DC bus precharge/RConn1 -- +VH/RConn1 -- DC/DC Boost Converter/RConn1

== system power_FCHPS_MEA2/Fuel Cell Power Module (FCPM) ==
  Bus Selector : BusSelector  OutputSignals=Voltage,Current,Stack consumption (lpm) [Air(Yellow); Fuel(Magenta)],Flow Rate (lpm [Air(Yellow); Fuel(Magenta)]  OutputAsBus=on
  Contactors1 : Subsystem
  FCPM Controller : Subsystem
  Fuel Cell Stack : electricdrivelib/Extra Sources/Fuel Cell Stack  PresetModel=No (User-Defined)  FcType=Proton Exchange Membrane (PEM)  Detailed=Detailed  Eoc="[52.5        52.46]"  NomVI="[250         41.15]"  EndVI="[320          39.2]"  Nc=65  n=50  TOp=45  AirFr=732  SuppPress="[1.16           1]"  Comp="[99.95           21            1]"  SignX=off  SignY=off  FlowRateH2=on  FlowRateAir=on  SystemTemp=off  SystemPH2=off  SystemPAir=off  FCDyn=on  FC_tau=1  Peak_O2=60  V_Under=2
      settings: SourceProductName=Simscape Power Systems  SourceProductBaseCode=PS
  Mux : Mux  Inputs=2
  Scope : Scope
  Scope1 : Scope
  Voltage Measurement : powerlib/Measurements/Voltage Measurement  PhasorSimulation=off  OutputType=Complex  PSBequivalent=0
  +VFC : PMIOPort  Port=1  Side=Right
  -VFC : PMIOPort  Port=2  Side=Right
  Mesures : Outport
  tag scope: Vfc=global
  wires:
  FCPM Controller/3(H2Fr) -> Fuel Cell Stack/1
  FCPM Controller/2(AirFr) -> Fuel Cell Stack/2
  Fuel Cell Stack/1 -> FCPM Controller/1(IFC), Bus Selector/1
  FCPM Controller/1(IFCmax) -> Mux/1
  Bus Selector/1 -> Mux/2
  Mux/1 -> Scope/1, Mesures/1
  Voltage Measurement/1 -> Scope1/1, [Vfc]
  connections:
  Contactors1/LConn1 -- Fuel Cell Stack/RConn1
  Voltage Measurement/LConn1 -- +VFC/RConn1 -- Contactors1/RConn1
  -VFC/RConn1 -- Fuel Cell Stack/RConn2 -- Voltage Measurement/LConn2

== system power_FCHPS_MEA2/Mesures 2 ==
  Current Measurement2 : powerlib/Measurements/Current Measurement  PhasorSimulation=off  OutputType=Complex  PSBequivalent=0
  Mux1 : Mux  Inputs=2
  Scope : Scope
  Scope1 : Scope
  Voltage Measurement2 : powerlib/Measurements/Voltage Measurement  PhasorSimulation=off  OutputType=Complex  PSBequivalent=0
  +M : PMIOPort  Port=1  Side=Left
  O : PMIOPort  Port=2  Side=Right
  -M : PMIOPort  Port=3  Side=Left
  M : Outport
  wires:
  Voltage Measurement2/1 -> Scope/1, Mux1/2
  Current Measurement2/1 -> Mux1/1
  Mux1/1 -> Scope1/1, M/1
  connections:
  +M/RConn1 -- Current Measurement2/LConn1
  -M/RConn1 -- Voltage Measurement2/LConn2
  Current Measurement2/RConn1 -- O/RConn1 -- Voltage Measurement2/LConn1

== system power_FCHPS_MEA2/Mesures1 ==
  Current Measurement2 : powerlib/Measurements/Current Measurement  PhasorSimulation=off  OutputType=Complex  PSBequivalent=0
  Mux1 : Mux  Inputs=2
  Scope : Scope
  Scope1 : Scope
  Voltage Measurement2 : powerlib/Measurements/Voltage Measurement  PhasorSimulation=off  OutputType=Complex  PSBequivalent=0
  +M : PMIOPort  Port=1  Side=Left
  O : PMIOPort  Port=2  Side=Right
  -M : PMIOPort  Port=3  Side=Left
  M : Outport
  wires:
  Mux1/1 -> Scope1/1, M/1
  Current Measurement2/1 -> Mux1/1
  Voltage Measurement2/1 -> Scope/1, Mux1/2
  connections:
  Voltage Measurement2/LConn1 -- O/RConn1 -- Current Measurement2/RConn1
  -M/RConn1 -- Voltage Measurement2/LConn2
  +M/RConn1 -- Current Measurement2/LConn1

== system power_FCHPS_MEA2/More Info ==

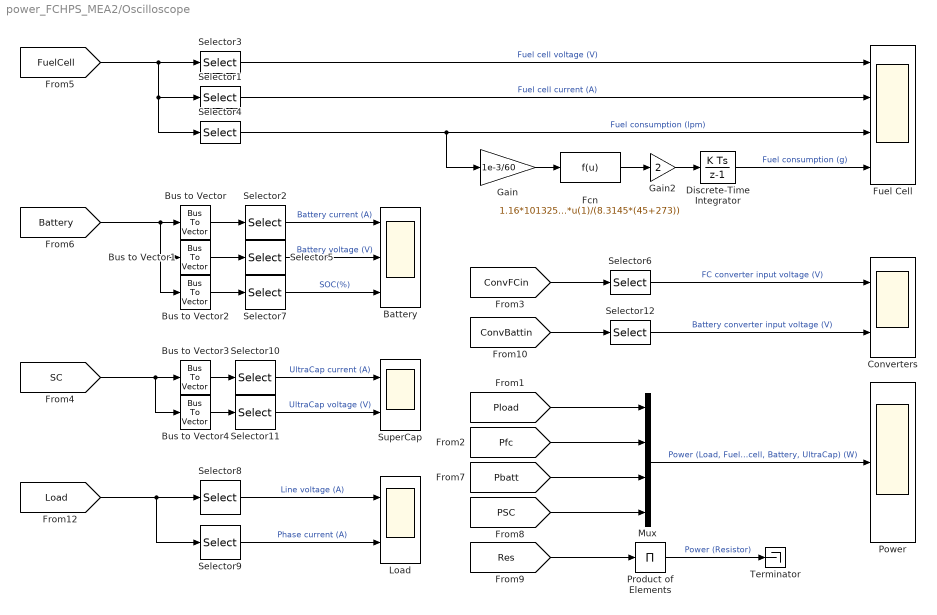
== system power_FCHPS_MEA2/Oscilloscope ==
  Battery : Scope  NumInputPorts=3
  Bus to Vector{,1..4} (5 alike) : BusToVector
  Converters : Scope  NumInputPorts=2
  Discrete-Time Integrator : DiscreteIntegrator  SampleTime=Ts  ICPrevOutput=DiscIntNeverNeededParam  ICPrevScaledInput=DiscIntNeverNeededParam
  Fcn : Fcn  Expr=1.16*101325*u(1)/(8.3145*(45+273))
  Fuel Cell : Scope  NumInputPorts=4
  Gain : Gain  Gain=1e-3/60
  Gain2 : Gain  Gain=2
  Load : Scope  NumInputPorts=2
  Mux : Mux
  Power : Scope
  Product of Elements : Product  Inputs=*
  Selector1 : Selector  InputPortWidth=7  IndexOptions=Index vector (dialog)  Indices=3  OutputSizes=1
  Selector10 : Selector  InputPortWidth=3  IndexOptions=Index vector (dialog)  Indices=[1]  OutputSizes=1
  Selector11 : Selector  InputPortWidth=3  IndexOptions=Index vector (dialog)  Indices=[2]  OutputSizes=1
  Selector12 : Selector  InputPortWidth=2  IndexOptions=Index vector (dialog)  Indices=2  OutputSizes=1
  Selector2 : Selector  InputPortWidth=3  IndexOptions=Index vector (dialog)  Indices=[2]  OutputSizes=1
  Selector3 : Selector  InputPortWidth=7  IndexOptions=Index vector (dialog)  Indices=2  OutputSizes=1
  Selector4 : Selector  InputPortWidth=7  IndexOptions=Index vector (dialog)  Indices=5  OutputSizes=1
  Selector5 : Selector  InputPortWidth=3  IndexOptions=Index vector (dialog)  Indices=[3]  OutputSizes=1
  Selector6 : Selector  InputPortWidth=2  IndexOptions=Index vector (dialog)  Indices=2  OutputSizes=1
  Selector7 : Selector  InputPortWidth=3  IndexOptions=Index vector (dialog)  Indices=[1]  OutputSizes=1
  Selector8 : Selector  InputPortWidth=6  IndexOptions=Index vector (dialog)  Indices=[1]  OutputSizes=1
  Selector9 : Selector  InputPortWidth=6  IndexOptions=Index vector (dialog)  Indices=4  OutputSizes=1
  SuperCap : Scope  NumInputPorts=2
  Terminator : Terminator
  wires:
  Selector1/1 -> Fuel Cell/2  "Fuel cell current (A)"
  Selector3/1 -> Fuel Cell/1  "Fuel cell voltage (V)"
  [FuelCell] -> Selector3/1, Selector1/1, Selector4/1
  Selector5/1 -> Battery/2  "Battery voltage (V)"
  Selector2/1 -> Battery/1  "Battery current (A)"
  [Battery] -> Bus to Vector/1, Bus to Vector1/1, Bus to Vector2/1
  Selector11/1 -> SuperCap/2  "UltraCap voltage (V)"
  Selector10/1 -> SuperCap/1  "UltraCap current (A)"
  [SC] -> Bus to Vector4/1, Bus to Vector3/1
  Mux/1 -> Power/1  "Power (Load, Fuel cell, Battery, UltraCap) (W)"
  Selector7/1 -> Battery/3  "SOC(%)"
  [Load] -> Selector9/1, Selector8/1
  Selector4/1 -> Gain/1, Fuel Cell/3  "Fuel consumption (lpm)"
  [Pload] -> Mux/1
  [Pfc] -> Mux/2
  [Pbatt] -> Mux/3
  [PSC] -> Mux/4
  Gain/1 -> Fcn/1
  Fcn/1 -> Gain2/1
  Discrete-Time Integrator/1 -> Fuel Cell/4  "Fuel consumption (g)"
  Gain2/1 -> Discrete-Time Integrator/1
  Selector8/1 -> Load/1  "Line voltage (A)"
  Selector9/1 -> Load/2  "Phase current (A)"
  [ConvFCin] -> Selector6/1
  [ConvBattin] -> Selector12/1
  Selector6/1 -> Converters/1  "FC converter input voltage (V)"
  Selector12/1 -> Converters/2  "Battery converter input voltage (V)"
  Product of Elements/1 -> Terminator/1  "Power (Resistor)"
  [Res] -> Product of Elements/1
  Bus to Vector/1 -> Selector2/1
  Bus to Vector1/1 -> Selector5/1
  Bus to Vector2/1 -> Selector7/1
  Bus to Vector3/1 -> Selector10/1
  Bus to Vector4/1 -> Selector11/1

== system power_FCHPS_MEA2/Protecting Resistor ==
  g : Inport
  Current Measurement : powerlib/Measurements/Current Measurement  PhasorSimulation=off  OutputType=Complex  PSBequivalent=0
  Ideal Switch : powerlib/Power Electronics/Ideal Switch  Ron=0.001  Lon=0  IC=0  Rs=10e3  Cs=inf  Measurements=off
  Mux : Mux  Inputs=2
  Series RLC Branch : powerlib/Elements/Series RLC Branch  LConnTagsString=__new0  RConnTagsString=__new0  BranchType=R  Resistance=6  Inductance=1e-3  SetiL0=off  InitialCurrent=0  Capacitance=1e-6  Setx0=off  InitialVoltage=0  Measurements=None
  Voltage Measurement : powerlib/Measurements/Voltage Measurement  PhasorSimulation=off  OutputType=Complex  PSBequivalent=0
  A : PMIOPort  Port=1  Side=Right
  B : PMIOPort  Port=2  Side=Right
  Mesures : Outport
  wires:
  g/1 -> Ideal Switch/1
  Current Measurement/1 -> Mux/1
  Voltage Measurement/1 -> Mux/2
  Mux/1 -> Mesures/1
  connections:
  Series RLC Branch/LConn1 -- Ideal Switch/LConn1
  B/RConn1 -- Series RLC Branch/RConn1 -- Voltage Measurement/LConn2
  Current Measurement/RConn1 -- Ideal Switch/RConn1
  Current Measurement/LConn1 -- A/RConn1 -- Voltage Measurement/LConn1

== system power_FCHPS_MEA2/3-phase AC load 功率可控的三相恒功率负载/Dynamic Impedance ==
  S : Inport
  pf : Inport  Port=2
  Fcn3 : Fcn  Expr=(sqrt(u(2)^2-u(1)^2))
  Fcn5 : Fcn  Expr=u(1)*u(2)
  Gain1 : Gain  Gain=2e3
  Gain3 : Gain  Gain=2e3
  Impedance Calculation : Subsystem
  Mux1 : Mux  Inputs=2
  Mux3 : Mux  Inputs=2
  Real-Imag to Complex1 : RealImagToComplex
  Z : Outport
  wires:
  Gain1/1 -> Real-Imag to Complex1/1
  Gain3/1 -> Real-Imag to Complex1/2
  Real-Imag to Complex1/1 -> Impedance Calculation/1(S)
  Impedance Calculation/1(Z) -> Z/1
  Mux1/1 -> Fcn5/1
  pf/1 -> Mux1/2
  Fcn5/1 -> Mux3/1, Gain1/1
  Mux3/1 -> Fcn3/1
  Fcn3/1 -> Gain3/1
  S/1 -> Mux1/1, Mux3/2

== system power_FCHPS_MEA2/DC//AC Converter/Control open loop1 ==
  Uabc Ref1 : Sin  Amplitude=VL*sqrt(2)  Frequency=2*pi*f  Phase="[0  2*pi/3  -2*pi/3]"  SampleTime=Ts
  g : Outport
  wires:
  Uabc Ref1/1 -> g/1
